simulink model "Problem_4"  (R2020b)
settings: Solver=ode45  StartTime=0.0  StopTime=10.0  RelTol=1e-3
values from neighbouring files (symbols this model uses):
  b = 3.5077E-6    (= 3.5077e-06)    [Parameters.m]
  J = 3.2284E-6    (= 3.2284e-06)    [Parameters.m]
  K = 0.0274    [Parameters.m]
  Kd = 0.489767517465838    (= 0.489767517466)    [Parameters.m]
  Ki = 4810.14360766501    (= 4810.14360767)    [Parameters.m]
  Kp = 97.1186920193705    (= 97.1186920194)    [Parameters.m]
  L = 2.75E-6    (= 2.75e-06)    [Parameters.m]
  n = 119827.875340723    (= 119827.875341)    [Parameters.m]
  R = 4    [Parameters.m]
settings Model: Creator=sansh  LastModifiedBy=adity
settings DataIOCC: ReturnWorkspaceOutputs=off
settings DebuggingCC: ArithmeticOperatorsInVariantConditions=warning
settings SFSimCC: SimUseLocalCustomCode=off  CustomCodeUndefinedFunction=UseInterfaceOnly
settings RTWCC: RTWUseLocalCustomCode=off
settings CodeAppCC: StateflowObjectComments=on

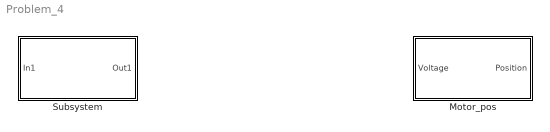
== system Problem_4 ==
  Motor_pos : Subsystem
  Subsystem : Subsystem

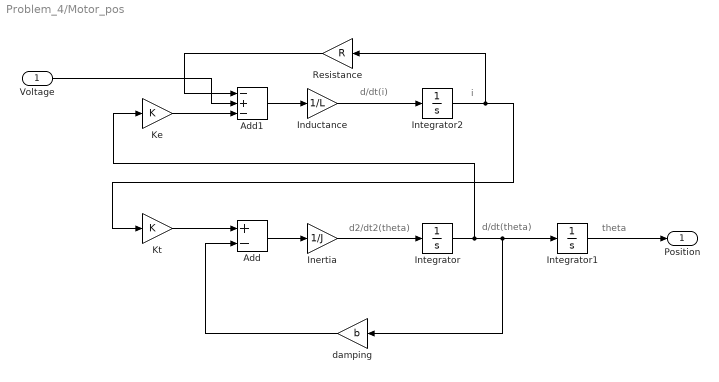
== system Problem_4/Motor_pos ==
  note: i
  note: d/dt(i)
  note: d2/dt2(theta)
  note: d/dt(theta)
  note: theta
  Voltage : Inport
  Add : Sum  Inputs=+-
  Add1 : Sum  Inputs=-+-
  Inductance : Gain  Gain=1/L
  Inertia : Gain  Gain=1/J
  Integrator : Integrator
  Integrator1 : Integrator
  Integrator2 : Integrator
  Ke : Gain  Gain=K
  Kt : Gain  Gain=K
  Resistance : Gain  Gain=R
  damping : Gain  Gain=b
  Position : Outport
  wires:
  Inertia/1 -> Integrator/1
  Inductance/1 -> Integrator2/1
  Integrator2/1 -> Resistance/1, Kt/1
  Integrator/1 -> Ke/1, damping/1, Integrator1/1
  Integrator1/1 -> Position/1
  Voltage/1 -> Add1/2
  Add/1 -> Inertia/1
  damping/1 -> Add/2
  Kt/1 -> Add/1
  Resistance/1 -> Add1/1
  Ke/1 -> Add1/3
  Add1/1 -> Inductance/1

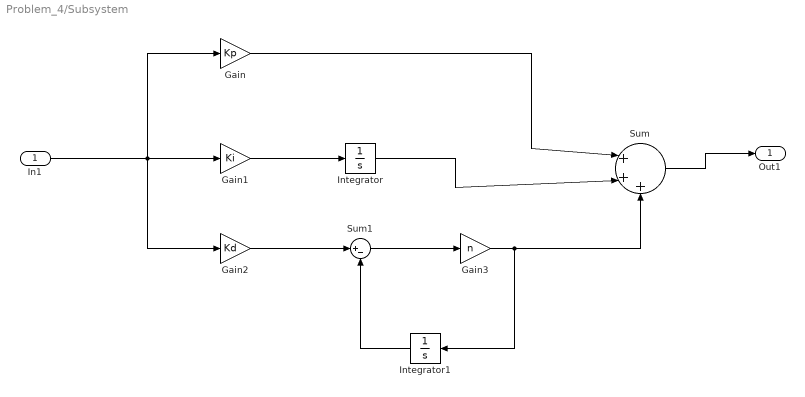
== system Problem_4/Subsystem ==
  In1 : Inport
  Gain : Gain  Gain=Kp
  Gain1 : Gain  Gain=Ki
  Gain2 : Gain  Gain=Kd
  Gain3 : Gain  Gain=n
  Integrator : Integrator
  Integrator1 : Integrator
  Sum : Sum  Inputs=|+++
  Sum1 : Sum  Inputs=|+-
  Out1 : Outport
  wires:
  Sum1/1 -> Gain3/1
  Gain2/1 -> Sum1/1
  Integrator1/1 -> Sum1/2
  Gain/1 -> Sum/1
  In1/1 -> Gain2/1, Gain/1, Gain1/1
  Gain1/1 -> Integrator/1
  Integrator/1 -> Sum/2
  Gain3/1 -> Sum/3, Integrator1/1
  Sum/1 -> Out1/1
